simulink model "CACC_4_Robots_Example_Cases"  (R2021a)
settings: Solver=FixedStepAuto  StartTime=0.0  StopTime=Tsim  RelTol=1e-3
values from neighbouring files (symbols this model uses):
  cIN = 0    [ros_cacc.m]    (also in ros_cacc2.m = 4)
  h = 1.0    (= 1)    [ros_cacc.m]    (also in ros_cacc2.m)
  k1 = 1    [ros_cacc.m]    (also in ros_cacc2.m)
  k2 = 1    [ros_cacc.m]    (also in ros_cacc2.m)
  r = 1    [ros_cacc.m]    (also in ros_cacc2.m)
  v_0 = 0.5    [ros_cacc.m]    (also in ros_cacc2.m)
  v_threshold = v_thr    (= 0.1)    [ros_cacc.m]    (also in ros_cacc2.m)
undefined symbols (not defined in the file or in its folder): angular, linear, sigbuilder_block
libraries: ros2lib x23, robotcorelib x4
(part 3 of 3)

== system CACC_4_Robots_Example_Cases/Subsystem2/controllers/Switch Case Ext. LA/disturbance term simplified/R(alph) ==
  In1 : Inport
  Bus Selector : BusSelector  OutputSignals=alpha
  R11 : Fcn  Expr=cos(u(1))
  R12 : Fcn  Expr=-sin(u(1))
  R21 : Fcn  Expr=sin(u(1))
  R22 : Fcn  Expr=cos(u(1))
  Vector Concatenate6 : Concatenate
  Vector Concatenate7 : Concatenate
  Vector Concatenate8 : Concatenate  Mode=Multidimensional array  ConcatenateDimension=2
  Out1 : Outport  VectorParamsAs1DForOutWhenUnconnected=off
  wires:
  Vector Concatenate8/1 -> Out1/1
  R22/1 -> Vector Concatenate7/2
  R12/1 -> Vector Concatenate7/1
  R21/1 -> Vector Concatenate6/2
  R11/1 -> Vector Concatenate6/1
  Vector Concatenate7/1 -> Vector Concatenate8/2
  Vector Concatenate6/1 -> Vector Concatenate8/1
  Bus Selector/1 -> R22/1, R21/1, R12/1, R11/1  "<alpha>"
  In1/1 -> Bus Selector/1

== system CACC_4_Robots_Example_Cases/Subsystem2/controllers/Switch Case Ext. LA/disturbance term simplified/beta1 ==
  In1 : Inport
  1 : Fcn  Expr=u(1)*cos(u(2))
  11 : Fcn  Expr=u(2)*(r+h*u(1))*sin(u(3))
  12 : Fcn  Expr=-sin(u(3))
  2 : Fcn  Expr=u(1)*sin(u(2))
  Bus Selector : BusSelector  OutputSignals=v,curv,alpha  OutputAsBus=on
  Bus Selector1 : BusSelector  OutputSignals=v_ref,theta_ref  OutputAsBus=on
  Product : Product  Multiplication=Matrix(*)
  Vector Concatenate : Concatenate
  Vector Concatenate1 : Concatenate
  Vector Concatenate2 : Concatenate  Mode=Multidimensional array  ConcatenateDimension=2
  Vector Concatenate3 : Concatenate
  Out1 : Outport  VectorParamsAs1DForOutWhenUnconnected=off
  wires:
  In1/1 -> Bus Selector1/1, Bus Selector/1
  Bus Selector/1 -> 11/1, 12/1
  11/1 -> Vector Concatenate1/2, Vector Concatenate/1
  12/1 -> Vector Concatenate1/1, Vector Concatenate/2
  Vector Concatenate/1 -> Vector Concatenate2/1
  Vector Concatenate1/1 -> Vector Concatenate2/2
  1/1 -> Vector Concatenate3/1
  2/1 -> Vector Concatenate3/2
  Bus Selector1/1 -> 2/1, 1/1
  Vector Concatenate2/1 -> Product/1
  Vector Concatenate3/1 -> Product/2
  Product/1 -> Out1/1

== system CACC_4_Robots_Example_Cases/Subsystem2/controllers/Switch Case Ext. LA/dz3,dz4 calculation/GamInv  ==
  In1 : Inport
  11 : Fcn  Expr=(r+h*u(1))*cos(u(2))
  12 : Fcn  Expr=(r+h*u(1))*sin(u(2))
  21 : Fcn  Expr=-h*sin(u(2))-h*sin(u(13))*cos(u(8))
  22 : Fcn  Expr=h*cos(u(2))-h*sin(u(13))*sin(u(8))
  Divide{,1..3} (4 alike) : Product  Inputs=*/
  Vector Concatenate : Concatenate
  Vector Concatenate1 : Concatenate
  Vector Concatenate2 : Concatenate  Mode=Multidimensional array  ConcatenateDimension=2
  det(Gam) : Fcn  Expr=((r+h*u(1))*(h-h*sin(u(13))*sin(u(8)-u(2))))
  GamInv : Outport  VectorParamsAs1DForOutWhenUnconnected=off
  wires:
  11/1 -> Divide/1
  12/1 -> Divide1/1
  21/1 -> Divide2/1
  22/1 -> Divide3/1
  det(Gam)/1 -> Divide2/2, Divide1/2, Divide/2, Divide3/2
  In1/1 -> det(Gam)/1, 22/1, 21/1, 12/1, 11/1
  Divide/1 -> Vector Concatenate/1
  Divide2/1 -> Vector Concatenate/2
  Divide1/1 -> Vector Concatenate1/1
  Divide3/1 -> Vector Concatenate1/2
  Vector Concatenate/1 -> Vector Concatenate2/1
  Vector Concatenate1/1 -> Vector Concatenate2/2
  Vector Concatenate2/1 -> GamInv/1

== system CACC_4_Robots_Example_Cases/Subsystem2/controllers/Switch Case Ext. LA/dz3,dz4 calculation/H_i ==
  In1 : Inport
  Bus Selector1 : BusSelector  OutputSignals=v,theta  OutputAsBus=on
  H11 : Fcn  Expr=cos(u(2))
  H12 : Fcn  Expr=-u(1)*sin(u(2))
  H21 : Fcn  Expr=sin(u(2))
  H22 : Fcn  Expr=u(1)*cos(u(2))
  Vector Concatenate3 : Concatenate
  Vector Concatenate4 : Concatenate
  Vector Concatenate5 : Concatenate  Mode=Multidimensional array  ConcatenateDimension=2
  Out1 : Outport  VectorParamsAs1DForOutWhenUnconnected=off
  wires:
  Bus Selector1/1 -> H11/1, H22/1, H21/1, H12/1
  In1/1 -> Bus Selector1/1
  Vector Concatenate3/1 -> Vector Concatenate5/1
  Vector Concatenate4/1 -> Vector Concatenate5/2
  H11/1 -> Vector Concatenate3/1
  H21/1 -> Vector Concatenate3/2
  H12/1 -> Vector Concatenate4/1
  H22/1 -> Vector Concatenate4/2
  Vector Concatenate5/1 -> Out1/1

== system CACC_4_Robots_Example_Cases/Subsystem2/controllers/Switch Case Ext. LA/dz3,dz4 calculation/H_i-1 ==
  In1 : Inport
  Bus Selector1 : BusSelector  OutputSignals=v_ref,theta_ref  OutputAsBus=on
  H11 : Fcn  Expr=cos(u(2))
  H12 : Fcn  Expr=-u(1)*sin(u(2))
  H21 : Fcn  Expr=sin(u(2))
  H22 : Fcn  Expr=u(1)*cos(u(2))
  Vector Concatenate3 : Concatenate
  Vector Concatenate4 : Concatenate
  Vector Concatenate5 : Concatenate  Mode=Multidimensional array  ConcatenateDimension=2
  Out1 : Outport  VectorParamsAs1DForOutWhenUnconnected=off
  wires:
  Vector Concatenate5/1 -> Out1/1
  H22/1 -> Vector Concatenate4/2
  H12/1 -> Vector Concatenate4/1
  H21/1 -> Vector Concatenate3/2
  H11/1 -> Vector Concatenate3/1
  Vector Concatenate4/1 -> Vector Concatenate5/2
  Vector Concatenate3/1 -> Vector Concatenate5/1
  In1/1 -> Bus Selector1/1
  Bus Selector1/1 -> H12/1, H21/1, H22/1, H11/1

== system CACC_4_Robots_Example_Cases/Subsystem2/controllers/Switch Case Ext. LA/dz3,dz4 calculation/R(alph) ==
  In1 : Inport
  Bus Selector : BusSelector  OutputSignals=alpha
  R11 : Fcn  Expr=cos(u(1))
  R12 : Fcn  Expr=-sin(u(1))
  R21 : Fcn  Expr=sin(u(1))
  R22 : Fcn  Expr=cos(u(1))
  Vector Concatenate6 : Concatenate
  Vector Concatenate7 : Concatenate
  Vector Concatenate8 : Concatenate  Mode=Multidimensional array  ConcatenateDimension=2
  Out1 : Outport  VectorParamsAs1DForOutWhenUnconnected=off
  wires:
  In1/1 -> Bus Selector/1
  Bus Selector/1 -> R11/1, R12/1, R21/1, R22/1  "<alpha>"
  Vector Concatenate6/1 -> Vector Concatenate8/1
  Vector Concatenate7/1 -> Vector Concatenate8/2
  R11/1 -> Vector Concatenate6/1
  R21/1 -> Vector Concatenate6/2
  R12/1 -> Vector Concatenate7/1
  R22/1 -> Vector Concatenate7/2
  Vector Concatenate8/1 -> Out1/1

== system CACC_4_Robots_Example_Cases/Subsystem2/controllers/Switch Case Ext. LA/dz3,dz4 calculation/Rinv(alph) ==
  In1 : Inport
  Bus Selector : BusSelector  OutputSignals=alpha
  R11 : Fcn  Expr=cos(u(1))
  R12 : Fcn  Expr=sin(u(1))
  R21 : Fcn  Expr=-sin(u(1))
  R22 : Fcn  Expr=cos(u(1))
  Vector Concatenate6 : Concatenate
  Vector Concatenate7 : Concatenate
  Vector Concatenate8 : Concatenate  Mode=Multidimensional array  ConcatenateDimension=2
  Out1 : Outport  VectorParamsAs1DForOutWhenUnconnected=off
  wires:
  Vector Concatenate8/1 -> Out1/1
  R22/1 -> Vector Concatenate7/2
  R12/1 -> Vector Concatenate7/1
  R21/1 -> Vector Concatenate6/2
  R11/1 -> Vector Concatenate6/1
  Vector Concatenate7/1 -> Vector Concatenate8/2
  Vector Concatenate6/1 -> Vector Concatenate8/1
  Bus Selector/1 -> R22/1, R21/1, R12/1, R11/1  "<alpha>"
  In1/1 -> Bus Selector/1

== system CACC_4_Robots_Example_Cases/Subsystem2/controllers/Switch Case Ext. LA/dz3,dz4 calculation/beta1 ==
  In1 : Inport
  Add : Sum
  Bus Selector2 : BusSelector  OutputSignals=alpha,v_ref,theta_ref  OutputAsBus=on
  Bus Selector3 : BusSelector  OutputSignals=theta_ref,thetadot_ref,s  OutputAsBus=on
  Fcn2 : Fcn  Expr=(1-cos(u(1)))*u(2)*cos(u(3))-sin(u(1))*u(2)*sin(u(3))
  Fcn3 : Fcn  Expr=sin(u(1))*u(2)*cos(u(3))+(1-cos(u(1)))*u(2)*sin(u(3))
  Fcn4 : Fcn  Expr=cos(u(1))*u(3)*u(2)
  Fcn5 : Fcn  Expr=sin(u(1))*u(3)*u(2)
  Mux3 : Mux  Inputs=2
  Mux4 : Mux  Inputs=2
  Out1 : Outport  VectorParamsAs1DForOutWhenUnconnected=off
  wires:
  Bus Selector2/1 -> Fcn3/1, Fcn2/1
  Fcn2/1 -> Mux3/1
  Fcn3/1 -> Mux3/2
  Bus Selector3/1 -> Fcn5/1, Fcn4/1
  Fcn4/1 -> Mux4/1
  Fcn5/1 -> Mux4/2
  Mux3/1 -> Add/1
  Mux4/1 -> Add/2
  In1/1 -> Bus Selector3/1, Bus Selector2/1
  Add/1 -> Out1/1

== system CACC_4_Robots_Example_Cases/Subsystem2/controllers/Switch Case Ext. LA/dz3,dz4 calculation/beta2 ==
  In1 : Inport
  Bus Selector : BusSelector  OutputSignals=v,theta,alpha,curv  OutputAsBus=on
  Mux : Mux  Inputs=2
  beta2_1 : Fcn  Expr=-u(1)*sin(u(2)+u(3))*(h*u(4)*cos(u(3))^2)
  beta2_2 : Fcn  Expr=u(1)*cos(u(2)+u(3))*(h*u(4)*cos(u(3))^2)
  Out1 : Outport  VectorParamsAs1DForOutWhenUnconnected=off
  wires:
  In1/1 -> Bus Selector/1
  Bus Selector/1 -> beta2_2/1, beta2_1/1
  beta2_1/1 -> Mux/1
  beta2_2/1 -> Mux/2
  Mux/1 -> Out1/1

== system CACC_4_Robots_Example_Cases/Subsystem2/controllers/Switch Case Ext. LA/dz3,dz4 calculation/eq Sig3 line 3 ==
  In1 : Inport
  1 : Fcn  Expr=u(1)*cos(u(2))
  2 : Fcn  Expr=u(1)*sin(u(2))
  Bus Selector1 : BusSelector  OutputSignals=v_ref,theta_ref  OutputAsBus=on
  Vector Concatenate3 : Concatenate
  mat : Subsystem
  Out1 : Outport  VectorParamsAs1DForOutWhenUnconnected=off
  v_i-1 : Outport  Port=2  VectorParamsAs1DForOutWhenUnconnected=off
  wires:
  In1/1 -> mat/1(In1), Bus Selector1/1
  Bus Selector1/1 -> 2/1, 1/1
  1/1 -> Vector Concatenate3/1
  2/1 -> Vector Concatenate3/2
  mat/1(Out1) -> Out1/1
  Vector Concatenate3/1 -> v_i-1/1

== system CACC_4_Robots_Example_Cases/Subsystem2/controllers/Switch Case Ext. LA/s/Approximation of s around zero ==
  In1 : Inport
  Action Port : ActionPort  ActionPortLabel=if(u1 < 0.01 & u1 > -0.01)
  Taylor approximation 3rd order : Fcn  Expr=0.5*(r+h*u(2))^2*u(1)-0.125*(r+h*u(2))^4*u(1)^3
  Out1 : Outport  VectorParamsAs1DForOutWhenUnconnected=off
  wires:
  In1/1 -> Taylor approximation 3rd order/1
  Taylor approximation 3rd order/1 -> Out1/1

== system CACC_4_Robots_Example_Cases/Subsystem2/controllers/Switch Case Ext. LA/s/function s ==
  In1 : Inport
  Action Port : ActionPort  ActionPortLabel=else
  function s : Fcn  Expr=(-1+sqrt(1+u(1)^2*(r+h*u(2))^2))/u(1)
  Out1 : Outport  VectorParamsAs1DForOutWhenUnconnected=off
  wires:
  In1/1 -> function s/1
  function s/1 -> Out1/1

== system CACC_4_Robots_Example_Cases/Subsystem/controllers/Switch Case Ext. LA/dz3,dz4 calculation/eq Sig3 line 3/mat ==
  In1 : Inport
  Bus Selector : BusSelector  OutputSignals=curv,v,alpha  OutputAsBus=on
  R11 : Fcn  Expr=u(1)*(r+h*u(2))*sin(u(3))
  R12 : Fcn  Expr=-sin(u(3))
  R21 : Fcn  Expr=sin(u(3))
  R22 : Fcn  Expr=u(1)*(r+h*u(2))*sin(u(3))
  Vector Concatenate6 : Concatenate
  Vector Concatenate7 : Concatenate
  Vector Concatenate8 : Concatenate  Mode=Multidimensional array  ConcatenateDimension=2
  Out1 : Outport  VectorParamsAs1DForOutWhenUnconnected=off
  wires:
  Vector Concatenate8/1 -> Out1/1
  R22/1 -> Vector Concatenate7/2
  R12/1 -> Vector Concatenate7/1
  R21/1 -> Vector Concatenate6/2
  R11/1 -> Vector Concatenate6/1
  Vector Concatenate7/1 -> Vector Concatenate8/2
  Vector Concatenate6/1 -> Vector Concatenate8/1
  Bus Selector/1 -> R12/1, R21/1, R22/1, R11/1
  In1/1 -> Bus Selector/1

== system CACC_4_Robots_Example_Cases/Subsystem1/controllers/Switch Case Ext. LA/dz3,dz4 calculation/eq Sig3 line 3/mat ==
  In1 : Inport
  Bus Selector : BusSelector  OutputSignals=curv,v,alpha  OutputAsBus=on
  R11 : Fcn  Expr=u(1)*(r+h*u(2))*sin(u(3))
  R12 : Fcn  Expr=-sin(u(3))
  R21 : Fcn  Expr=sin(u(3))
  R22 : Fcn  Expr=u(1)*(r+h*u(2))*sin(u(3))
  Vector Concatenate6 : Concatenate
  Vector Concatenate7 : Concatenate
  Vector Concatenate8 : Concatenate  Mode=Multidimensional array  ConcatenateDimension=2
  Out1 : Outport  VectorParamsAs1DForOutWhenUnconnected=off
  wires:
  Vector Concatenate8/1 -> Out1/1
  R22/1 -> Vector Concatenate7/2
  R12/1 -> Vector Concatenate7/1
  R21/1 -> Vector Concatenate6/2
  R11/1 -> Vector Concatenate6/1
  Vector Concatenate7/1 -> Vector Concatenate8/2
  Vector Concatenate6/1 -> Vector Concatenate8/1
  Bus Selector/1 -> R12/1, R21/1, R22/1, R11/1
  In1/1 -> Bus Selector/1

== system CACC_4_Robots_Example_Cases/Subsystem2/controllers/Switch Case Ext. LA/dz3,dz4 calculation/eq Sig3 line 3/mat ==
  In1 : Inport
  Bus Selector : BusSelector  OutputSignals=curv,v,alpha  OutputAsBus=on
  R11 : Fcn  Expr=u(1)*(r+h*u(2))*sin(u(3))
  R12 : Fcn  Expr=-sin(u(3))
  R21 : Fcn  Expr=sin(u(3))
  R22 : Fcn  Expr=u(1)*(r+h*u(2))*sin(u(3))
  Vector Concatenate6 : Concatenate
  Vector Concatenate7 : Concatenate
  Vector Concatenate8 : Concatenate  Mode=Multidimensional array  ConcatenateDimension=2
  Out1 : Outport  VectorParamsAs1DForOutWhenUnconnected=off
  wires:
  Vector Concatenate8/1 -> Out1/1
  R22/1 -> Vector Concatenate7/2
  R12/1 -> Vector Concatenate7/1
  R21/1 -> Vector Concatenate6/2
  R11/1 -> Vector Concatenate6/1
  Vector Concatenate7/1 -> Vector Concatenate8/2
  Vector Concatenate6/1 -> Vector Concatenate8/1
  Bus Selector/1 -> R12/1, R21/1, R22/1, R11/1
  In1/1 -> Bus Selector/1
